simulink model "BatterySOHEstimation"  (R2024a)
settings: Solver=VariableStepAuto  StartTime=0.0  StopTime=10*10000  FixedStep=Ts  RelTol=1e-3  EnableMultiTasking=on
PreLoadFcn:
  | BatterySOHEstimationData;
values from neighbouring files (symbols this model uses):
  R = 0.05    [BatterySOHEstimationData.m]
  R00 = 0.008    [BatterySOHEstimationData.m]
  R0_mat = [.0117, .0085, .009; .011, .0085, .009;     .0114, .0087, .0092; .0107, .0082, .0088; .0107, .0083, .0091;     .0113, .0085, .0089; .0116, .0085, .0089]    [BatterySOHEstimationData.m]
  SOC0 = initialSOC    (= 0.1)    [BatterySOHEstimationData.m]
  Ts = 1    [BatterySOHEstimationData.m]
libraries: fl_lib x8, nesl_utility x5, simulink x3, BatteryEstimators x2, batteryecm_lib x1
CloseFcn:
  | try
  |     close(h1_BatterySOHEstimation)
  | catch
  | end
  | 
  | clear h1_BatterySOHEstimation
  | 
  | clear BatterySOHEstimationSimlog
  | clear BatterySOHEstimationLogsout
  | 
  | clear AH SOC_vec T_vec R0_mat R1_mat tau1_mat
  | clear V0_mat Q R P0 initialSOC SOC0 R00 Ts
  | clear cell_area h_conv thermal_mass
Description:
  | Battery State-of-Health Estimation
settings Model: Creator=The MathWorks, Inc.  LastModifiedBy=Carlos
settings SolverCC: AlgebraicLoopSolver=TrustRegion  AutoInsertRateTranBlk=on  MaxZcPerStep=1
settings DataIOCC: MaxDataPoints=370000  ReturnWorkspaceOutputs=off  SignalLoggingName=BatterySOHEstimationLogsout
settings OptimizationCC: ReuseModelBlockBuffer=off  LifeSpan=inf
settings DebuggingCC: UnconnectedInputMsg=warning  UnconnectedOutputMsg=warning  UnconnectedLineMsg=warning  SFUnexpectedBacktrackingDiag=warning  SFNoUnconditionalDefaultTransitionDiag=warning  SFExecutionAtInitializationDiag=none  ArithmeticOperatorsInVariantConditions=warning
settings ModelReferenceCC: EnableRefExpFcnMdlSchedulingChecks=on
settings SFSimCC: SimUseLocalCustomCode=off  CustomCodeUndefinedFunction=UseInterfaceOnly
settings RTWCC: RTWUseLocalCustomCode=off  GPUComputeCapability=3.5  DLArmComputeVersion=19.05
settings CodeAppCC: StateflowObjectComments=on
settings GRTTargetCC: TargetLangStandard=C89/C90 (ANSI)
settings ConfigComp: CovMetricSettings=dw  CovSaveCumulativeToWorkspaceVar=on  CovSaveSingleToWorkspaceVar=on  CovExternalEMLEnable=off
settings SimscapeCC: SimscapeLogType=all  SimscapeLogSimulationStatistics=on  SimscapeLogName=BatterySOHEstimationSimlog  SimscapeLogDataHistory=370000

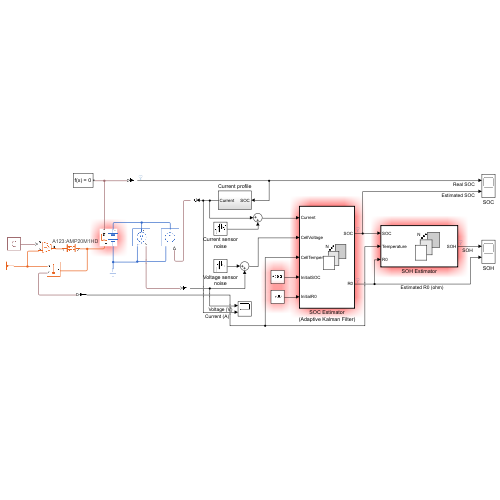
[thumbnail: Simulink's stored preview of the top-level diagram]
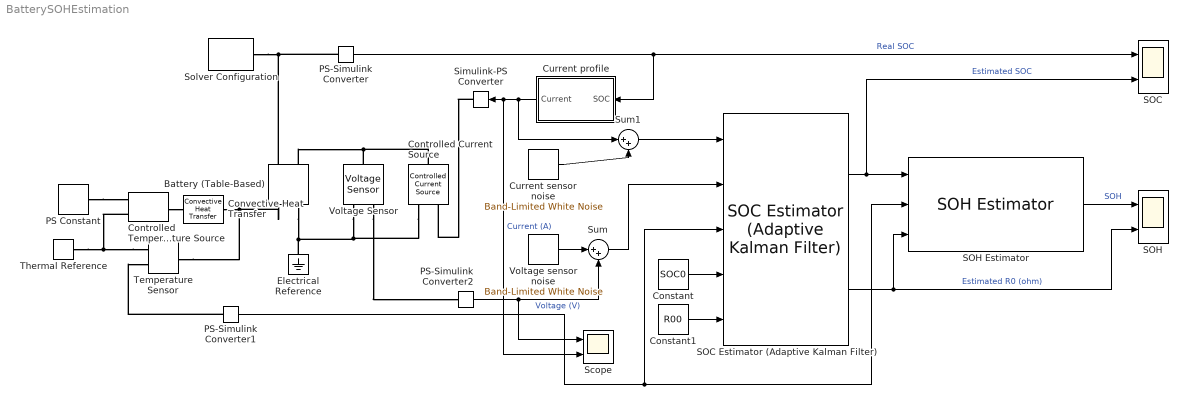
== system BatterySOHEstimation ==
  Battery (Table-Based) : batteryecm_lib/Battery (Table-Based)  Tag={'toolbox/physmod/battery/shared_library/m/batteryecm_lib_parts';'Battery__Table_Based_/A123/AMP20M1HD.xml'}  SOC_vec=SOC_vec  T_dependence=simscape.enum.tablebattery.temperature_dependence.yes  prm_dir=simscape.enum.tablebattery.prm_dir.noCurrentDirectionality  T_vec=T_vec K  V0_mat=V0_mat V  V0_vec=[2.93217 2.94263 2.95309 2.96355 2.97401 2.98447 2.99493 3.02455 3.05382 3.07377 3.08453 3.09529 3.09916 3.10271 3.10625 3.1098 3.11335 3.11689 3.12044 3.13089 3.13795 3.14459 3.14961 3.15451 3.15932 3.16324 3.16716 3.17063 3.17297 3.17544 3.17798 3.18052 3.18295 3.18533 3.18771 3.19009 3.19215 3.19403 3.1959 3.19777 3.1998 3.20198 3.20371 3.20501 3.20619 3.20738 3.20856 3.20974 3.21092 3.2121 3.21329 3.21447 3.21565 3.21672 3.21787 3.21904 3.22021 3.22139 3.22256 3.22374 3.22492 3.2261 3.22728 3.22847 3.22965 3.23083 3.23201 3.23319 3.23437 3.23552 3.23652 3.23778 3.23909 3.24045 3.24217 3.2439 3.24563 3.24736 3.24909 3.25082 3.25255 3.25428 3.256 3.25774 3.25951 3.26116 3.26238 3.26307 3.26352 3.26396 3.26441 3.26485 3.2653 3.26593 3.26612 3.26743 3.26879 3.27596 3.2842 3.30299 3.33677] V  V_range=[1.8 Inf] V  R0_mat=R0_mat Ohm  R0_vec=[0.00349 0.0033 0.00311 0.00292 0.00272 0.00253 0.00235 0.00233 0.00235 0.00232 0.00223 0.00214 0.00205 0.00196 0.00187 0.00181 0.00175 0.00169 0.00164 0.00167 0.00168 0.00168 0.00168 0.00168 0.00167 0.00167 0.00167 0.00167 0.00166 0.00165 0.00164 0.00164 0.00163 0.00163 0.00162 0.00162 0.00161 0.0016 0.00159 0.00159 0.00158 0.00158 0.00158 0.00157 0.00156 0.00156 0.00155 0.00154 0.00154 0.00153 0.00153 0.00152 0.00151 0.00151 0.0015 0.0015 0.0015 0.00149 0.00149 0.00149 0.00148 0.00148 0.00148 0.00147 0.00147 0.00147 0.00147 0.00146 0.00146 0.00146 0.00145 0.00146 0.00146 0.00147 0.00147 0.00148 0.00149 0.0015 0.0015 0.00151 0.00152 0.00153 0.00153 0.00154 0.00155 0.00155 0.00156 0.00155 0.00154 0.00153 0.00152 0.00151 0.0015 0.00148 0.00144 0.0014 0.00137 0.00136 0.00131 0.00127 0.00104] Ohm  R0_dis_mat=[.0117, .0085, .009; .011, .0085, .009; .0114, .0087, .0092; .0107, .0082, .0088; .0107, .0083, .0091; .0113, .0085, .0089; .0116, .0085, .0089] % Parameter not set Ohm  R0_dis_vec=[.0085, .0085, .0087, .0082, .0083, .0085, .0085] % Parameter not set Ohm  R0_ch_mat=[.0117, .0085, .009; .011, .0085, .009; .0114, .0087, .0092; .0107, .0082, .0088; .0107, .0083, .0091; .0113, .0085, .0089; .0116, .0085, .0089] % Parameter not set Ohm  R0_ch_vec=[.0085, .0085, .0087, .0082, .0083, .0085, .0085] % Parameter not set Ohm  AH=AH hr*A  prm_leak=simscape.enum.tablebattery.prm_leak.disabled  Rleak_vec=[8000, 7000, 6000] % Parameter not set Ohm  Rleak=7e3 % Parameter not set Ohm  extrapolation_option=simscape.enum.extrapolation.nearest  SOC_port=simscape.enum.tablebattery.enable.yes  prm_dyn=simscape.enum.tablebattery.prm_dyn.rc1  R1_mat=R1_mat Ohm  R1_vec=[.0029, .0024, .0026, .0016, .0023, .0018, .0017] % Parameter not set Ohm  tau1_mat=tau1_mat s  tau1_vec=[36, 45, 105, 29, 77, 33, 39] % Parameter not set s  R2_mat=[.0109, .0029, .0013; .0069, .0024, .0012; .0047, .0026, .0013; .0034, .0016, .001; .0033, .0023, .0014; .0033, .0018, .0011; .0028, .0017, .0011] % Parameter not set Ohm  R2_vec=[.0029, .0024, .0026, .0016, .0023, .0018, .0017] % Parameter not set Ohm  tau2_mat=[20, 36, 39; 31, 45, 39; 109, 105, 61; 36, 29, 26; 59, 77, 67; 40, 33, 29; 25, 39, 33] % Parameter not set s  tau2_vec=[36, 45, 105, 29, 77, 33, 39] % Parameter not set s  R3_mat=[.0109, .0029, .0013; .0069, .0024, .0012; .0047, .0026, .0013; .0034, .0016, .001; .0033, .0023, .0014; .0033, .0018, .0011; .0028, .0017, .0011] % Parameter not set Ohm  R3_vec=[.0029, .0024, .0026, .0016, .0023, .0018, .0017] % Parameter not set Ohm  tau3_mat=[20, 36, 39; 31, 45, 39; 109, 105, 61; 36, 29, 26; 59, 77, 67; 40, 33, 29; 25, 39, 33] % Parameter not set s  tau3_vec=[36, 45, 105, 29, 77, 33, 39] % Parameter not set s  R4_mat=[.0109, .0029, .0013; .0069, .0024, .0012; .0047, .0026, .0013; .0034, .0016, .001; .0033, .0023, .0014; .0033, .0018, .0011; .0028, .0017, .0011] % Parameter not set Ohm  R4_vec=[.0029, .0024, .0026, .0016, .0023, .0018, .0017] % Parameter not set Ohm  tau4_mat=[20, 36, 39; 31, 45, 39; 109, 105, 61; 36, 29, 26; 59, 77, 67; 40, 33, 29; 25, 39, 33] % Parameter not set s  tau4_vec=[36, 45, 105, 29, 77, 33, 39] % Parameter not set s  R5_mat=[.0109, .0029, .0013; .0069, .0024, .0012; .0047, .0026, .0013; .0034, .0016, .001; .0033, .0023, .0014; .0033, .0018, .0011; .0028, .0017, .0011] % Parameter not set Ohm  R5_vec=[.0029, .0024, .0026, .0016, .0023, .0018, .0017] % Parameter not set Ohm  tau5_mat=[20, 36, 39; 31, 45, 39; 109, 105, 61; 36, 29, 26; 59, 77, 67; 40, 33, 29; 25, 39, 33] % Parameter not set s  tau5_vec=[36, 45, 105, 29, 77, 33, 39] % Parameter not set s  prm_fade=simscape.enum.tablebattery.prm_fade.tableNandT  N0=100 % Parameter not set  dV0=0 % Parameter not set  dR0=0 % Parameter not set  dAH=0 % Parameter not set  dRleak=0 % Parameter not set  dR1=0 % Parameter not set  dR2=0 % Parameter not set  dR3=0 % Parameter not set  dR4=0 % Parameter not set  dR5=0 % Parameter not set  N0vec=N0vec  Tfadevec=Tfadevec K  dV0vec=[0 -0.3227 -0.6453 -0.9509 -1.1187 -1.2594 -1.4 -1.5407 -1.6219 -1.683 -1.7439 -1.8049 -1.8602 -1.9134 -1.9665 -2.0196 -2.0441 -2.0544 -2.0647 -2.075 -2.085 -2.0949 -2.1048 -2.1146 -2.1183 -2.1198 -2.1212 -2.1226 -2.1259 -2.1303 -2.1347 -2.1391 -2.1431 -2.1462 -2.1493 -2.1524 -2.1556 -2.1591 -2.1625 -2.166 -2.1695 -2.1729 -2.1764 -2.1798 -2.1833 -2.1867 -2.1902 -2.1936 -2.197 -2.2002 -2.2034 -2.2067 -2.2106 -2.2156 -2.2206 -2.2256 -2.2316 -2.2405 -2.2493 -2.2582 -2.2676 -2.2798 -2.292 -2.3042 -2.3164 -2.3294 -2.3424 -2.3556 -2.3688 -2.3818 -2.3947 -2.4077 -2.4207 -2.4336 -2.4465 -2.4594 -2.4722 -2.485 -2.4978 -2.5106 -2.5233 -2.5361 -2.5489 -2.5617 -2.5745 -2.5872 -2.5999 -2.6126 -2.6253 -2.6381 -2.6508 -2.6635 -2.6765 -2.6898 -2.703 -2.7163 -2.7295 -2.7428 -2.756 -2.7693]  dR0vec=[0 0 0 0 0 0 0 0 0 0 0 0 0 0 0 0 0 0 0 0 0 0 0 0 0 0 0 0 0 0 0 0 0 0 0 0 0 0 0 0 0 0 0 0 0 0 0 0 0 0 0 0 0 0 0 0 0 0 0 0 0 0 0 0 0 0 0 0 0 0 0 0 0 0 0 0 0 0 0 0 0 0 0 0 0 0 0 0 0 0 0 0 0 0 0 0 0 0 0 0] % Parameter assumed  dAHvec=[0 -0.319 -0.638 -0.939 -1.189 -1.439 -1.688 -1.938 -2.188 -2.435 -2.682 -2.93 -3.177 -3.424 -3.671 -3.918 -4.169 -4.421 -4.673 -4.925 -5.177 -5.429 -5.681 -5.933 -6.185 -6.437 -6.683 -6.917 -7.152 -7.386 -7.621 -7.855 -8.09 -8.324 -8.558 -8.793 -9.033 -9.292 -9.551 -9.809 -10.068 -10.327 -10.586 -10.845 -11.104 -11.363 -11.622 -11.88 -12.132 -12.374 -12.616 -12.857 -13.099 -13.341 -13.582 -13.824 -14.066 -14.307 -14.549 -14.791 -15.035 -15.281 -15.526 -15.772 -16.017 -16.263 -16.508 -16.757 -17.007 -17.256 -17.506 -17.755 -18.005 -18.254 -18.504 -18.752 -18.999 -19.246 -19.493 -19.74 -19.986 -20.233 -20.48 -20.727 -20.973 -21.219 -21.464 -21.71 -21.955 -22.201 -22.446 -22.692 -22.943 -23.199 -23.455 -23.711 -23.966 -24.222 -24.478 -24.733]  dRleakvec=[0, 0, 0, 0] % Parameter not set  dR1vec=[0, 0, 0, 0] % Parameter not set  dR2vec=[0, 0, 0, 0] % Parameter not set  dR3vec=[0, 0, 0, 0] % Parameter not set  dR4vec=[0, 0, 0, 0] % Parameter not set  dR5vec=[0, 0, 0, 0] % Parameter not set  dV0mat=dV0mat  dR0mat=dR0mat  dAHmat=dAHmat  dRleakmat=[0, 0; 0, 0; 0, 0; 0, 0] % Parameter not set  dR1mat=dR1mat  dR2mat=[0, 0; 0, 0; 0, 0; 0, 0] % Parameter not set  dR3mat=[0, 0; 0, 0; 0, 0; 0, 0] % Parameter not set  dR4mat=[0, 0; 0, 0; 0, 0; 0, 0] % Parameter not set  dR5mat=[0, 0; 0, 0; 0, 0; 0, 0] % Parameter not set  prm_age_modeling=simscape.enum.tablebattery.prm_age_modeling.tableTandTime  storage_dt_age_vec=storage_dt_age_vec d  storage_T_age_vec=storage_T_age_vec K  prm_age_OCV=simscape.enum.tablebattery.prm_age_OCV.OCV  OCV_age=0.9 % Parameter not set  SOC_age=0.6 % Parameter not set  prm_age_resistance=simscape.enum.tablebattery.prm_age.disabled  OCV_scaling_age_resistance=2.2134e6 % Parameter not set  OCV_offset_age_resistance=1.632e6 % Parameter not set  temp_exp_age_resistance=0.515833569 % Parameter not set V  t_exp_age_resistance=0.75 % Parameter not set  T_age_vec_resistance=[273.15, 298.15, 323.15] % Parameter not set K  dt_age_vec_resistance=[0, 90, 180, 270] % Parameter not set d  dR0_age_vec=[0, 0, 0] % Parameter not set  t_meas_dR0_age=100 % Parameter not set d  dR0_age_mat=[0, 0, 0; 0, 0, 0; 0, 0, 0; 0, 0, 0] % Parameter not set  prm_age_capacity=simscape.enum.tablebattery.prm_age.enabled  OCV_scaling_age_capacity=1.5097e07 % Parameter not set  OCV_offset_age_capacity=8.3625e06 % Parameter not set  temp_exp_age_capacity=0.6011 % Parameter not set V  t_exp_age_capacity=0.75 % Parameter not set  T_age_vec_capacity=T_age_vec_capacity K  dt_age_vec_capacity=dt_age_vec_capacity d  dAH_age_vec=[0, 0, 0] % Parameter not set  t_meas_dAH_age=100 % Parameter not set d  dAH_age_mat=dAH_age_mat  thermal_port=simscape.enum.thermaleffects.model  temperature=298.15 % Parameter not set K  thermal_mass=446.4 % Parameter assumed J/K  i_specify=on  i_priority=None  i=i A  i_nominal_specify=off  i_nominal_value=1  i_nominal_unit=A  v_specify=on  v_priority=None  v=v V  v_nominal_specify=on  v_nominal_value=v_nominal_value  v_nominal_unit=V  stateOfCharge_specify=on  stateOfCharge_priority=High  stateOfCharge=initialSOC  stateOfCharge_nominal_specify=on  stateOfCharge_nominal_value=finalSOC  stateOfCharge_nominal_unit=1  num_cycles_specify=on  num_cycles_priority=High  num_cycles=num_cycles  num_cycles_nominal_specify=on  num_cycles_nominal_value=num_cycles_nominal_value  num_cycles_nominal_unit=1  cell_temperature_specify=on  cell_temperature_priority=High  cell_temperature=cell_temperature K  cell_temperature_nominal_specify=off  cell_temperature_nominal_value=1  cell_temperature_nominal_unit=K
      settings: AttributesFormatString=A123:AMP20M1HD
  Constant : Constant  Value=SOC0
  Constant1 : Constant  Value=R00
  Controlled Temperature Source : fl_lib/Thermal/Thermal Sources/Controlled Temperature Source
  Controlled Current Source : fl_lib/Electrical/Electrical Sources/Controlled Current Source
  Convective Heat Transfer : fl_lib/Thermal/Thermal Elements/Convective Heat Transfer  thermal_type=foundation.enum.constant_variable.constant  area=0.1019 m^2  heat_tr_coeff=5 W/(K*m^2)  min_heat_tr_coeff=1e-3 W/(K*m^2)  T_specify=off  T_priority=None  T=0 K  T_nominal_specify=off  T_nominal_value=1  T_nominal_unit=K  Q_specify=off  Q_priority=None  Q=0 W  Q_nominal_specify=off  Q_nominal_value=1  Q_nominal_unit=W
  Current profile : Subsystem
  Current sensor noise : simulink/Sources/Band-Limited White Noise  Cov=1e-3  Ts=1  seed=1
  Electrical Reference : fl_lib/Electrical/Electrical Elements/Electrical Reference
  PS Constant : fl_lib/Physical Signals/Sources/PS Constant  constant=292.15 K
  PS-Simulink Converter : nesl_utility/PS-Simulink Converter  PhysicalDomain=network_engine_domain  SubClassName=ps_output  LeftPortType=input  RightPortType=output  PseudoPeriodic=off  Frequencies=[]  VectorFormat=inherit  Unit=inherit  AffineConversion=off
  PS-Simulink Converter1 : nesl_utility/PS-Simulink Converter  PhysicalDomain=network_engine_domain  SubClassName=ps_output  LeftPortType=input  RightPortType=output  PseudoPeriodic=off  Frequencies=[]  VectorFormat=inherit  Unit=inherit  AffineConversion=off
  PS-Simulink Converter2 : nesl_utility/PS-Simulink Converter  PhysicalDomain=network_engine_domain  SubClassName=ps_output  LeftPortType=input  RightPortType=output  PseudoPeriodic=off  Frequencies=[]  VectorFormat=inherit  Unit=inherit  AffineConversion=off
  SOC : Scope  NumInputPorts=2
  SOC Estimator (Adaptive Kalman Filter) : BatteryEstimators/SOC Estimator (Adaptive Kalman Filter)  CurrentInputPartition=off  filterType=Unscented Kalman filter  alpha=1  beta=2  kappa=0  Q=Q  Q_2RC=|  R=R  P0=P0  P0_2RC="[1e-5 0 0 0; 0 1 0 0;0 0  1 0; 0 0 0 1e-5]"  Ts=Ts  chargeDynamics=One time-constant dynamics  SOC_vec=SOC_vec  T_vec=T_vec  R1_mat=R1_mat  tau1_mat=tau1_mat  R2_mat=[.0109, .0029, .0013; .0069, .0024, .0012; .0047, .0026, .0013; .0034, .0016, .001; .0033, .0023, .0014; .0033, .0018, .0011; .0028, .0017, .0011]  tau2_mat=[20, 36, 39; 31, 45, 39; 109, 105, 61; 36, 29, 26; 59, 77, 67; 40, 33, 29; 25, 39, 33]  V0_mat=V0_mat  AH=AH
      | [1e-6 0 0 0;
      | 0 1e-6 0 0;0 0 1e-6 0;0 0 0 1e-6]
  SOH : Scope  NumInputPorts=2
  SOH Estimator : BatteryEstimators/SOH Estimator  SOC_vec=SOC_vec  T_vec=T_vec  R0_new_mat=R0_mat  R0_EOL_mat=R0_mat*3
  Scope : Scope  NumInputPorts=2
  Simulink-PS Converter : nesl_utility/Simulink-PS Converter  PhysicalDomain=network_engine_domain  SubClassName=ps_input  LeftPortType=input  RightPortType=output  PseudoPeriodic=off  Frequencies=[]  NoiseDistribution=none  NoiseParameters=[]  Unit=1  AffineConversion=off  FilteringAndDerivatives=provide  SimscapeFilterOrder=1  InputFilterTimeConstant=0.001  UdotUserProvided=0
  Solver Configuration : nesl_utility/Solver Configuration  PhysicalDomain=network_engine_domain  SubClassName=solver  LeftPortType=input  RightPortType=generic  Tones=[]  Harmonics=[]  SimulateNoise=off  Profile=off  UseLocalSampling=off  EnableSwitchedLinearOptims=on  FrequencyDomain=off  UseCCode=off  RelTol=0.001  AbsTol=0.001  MinStep=1e-09  ToWorkspace=off  RevertToSquareIcSolve=off  NumHomotopyIterations=100  PhasorMode=off  PhasorModeNumHarmonics=1  ConsistencySolver=NEWTON_XTOL_AFTER_FTOL  IndexReductionMethod=DerivativeReplacement  DoDC=off  ResidualTolerance=1e-09  ConsistencyTolSource=GLOBAL  ConsistencyAbsTol=0.001  ConsistencyRelTol=0.001  ConsistencyTolFactor=0.001  UseLocalSolver=off  LocalSolverChoice=NE_BACKWARD_EULER_ADVANCER  ResolveIndetEquations=on  FunctionEvalNumThread=1  LocalSolverSampleTime=0.001  DoFixedCost=off  MaxNonlinIter=3  MaxModeIter=2  ComputeImpulses=off  ImpulseIterations=2  LinearAlgebra=auto  LinearAlgebraNumThread=0  EquationFormulation=NE_TIME_EF  DelaysMemoryBudget=1024  AutomaticFiltering=on  FilteringTimeConstant=0.001  PartitionStorageMethod=AS_NEEDED  PartitionMemoryBudget=1024  PartitionMethod=ROBUST  MultibodyUseLocalSolver=off  MultibodyLocalSolverChoice=ODE1  MultibodyLocalSolverSampleTime=0.001
  Sum : Sum  Inputs=|++
  Sum1 : Sum  Inputs=|++
  Temperature Sensor : fl_lib/Thermal/Thermal Sensors/Temperature Sensor  temperature_measure=foundation.enum.MeasurementReference.difference
  Thermal Reference : fl_lib/Thermal/Thermal Elements/Thermal Reference
  Voltage Sensor : fl_lib/Electrical/Electrical Sensors/Voltage Sensor
  Voltage sensor noise : simulink/Sources/Band-Limited White Noise  Cov=1e-3  Ts=1  seed=23341
  wires:
  Sum1/1 -> SOC Estimator (Adaptive Kalman Filter)/1
  Sum/1 -> SOC Estimator (Adaptive Kalman Filter)/2
  PS-Simulink Converter1/1 -> SOH Estimator/2, SOC Estimator (Adaptive Kalman Filter)/3
  Constant/1 -> SOC Estimator (Adaptive Kalman Filter)/4
  Constant1/1 -> SOC Estimator (Adaptive Kalman Filter)/5
  SOC Estimator (Adaptive Kalman Filter)/1 -> SOH Estimator/1, SOC/2  "Estimated SOC"
  SOC Estimator (Adaptive Kalman Filter)/2 -> SOH/2, SOH Estimator/3  "Estimated R0 (ohm)"
  Current profile/1(Current) -> Sum1/1, Scope/2, Simulink-PS Converter/1  "Current (A)"
  PS-Simulink Converter/1 -> Current profile/1(SOC), SOC/1  "Real SOC"
  SOH Estimator/1 -> SOH/1  "SOH"
  Voltage sensor noise/1 -> Sum/1
  Current sensor noise/1 -> Sum1/2
  PS-Simulink Converter2/1 -> Scope/1, Sum/2  "Voltage (V)"
  connections:
  PS-Simulink Converter/LConn1 -- Battery (Table-Based)/LConn2 -- Solver Configuration/RConn1
  Electrical Reference/LConn1 -- Battery (Table-Based)/RConn1 -- Controlled Current Source/RConn2 -- Voltage Sensor/RConn2
  Voltage Sensor/LConn1 -- Battery (Table-Based)/LConn1 -- Controlled Current Source/LConn1
  Simulink-PS Converter/RConn1 -- Controlled Current Source/RConn1
  Voltage Sensor/RConn1 -- PS-Simulink Converter2/LConn1
  Temperature Sensor/LConn1 -- Battery (Table-Based)/RConn2 -- Convective Heat Transfer/LConn1
  Temperature Sensor/RConn1 -- Thermal Reference/LConn1 -- Controlled Temperature Source/RConn2
  Controlled Temperature Source/LConn1 -- Convective Heat Transfer/RConn1
  PS-Simulink Converter1/LConn1 -- Temperature Sensor/RConn2
  PS Constant/RConn1 -- Controlled Temperature Source/RConn1

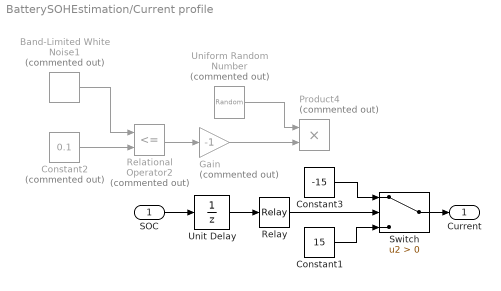
== system BatterySOHEstimation/Current profile ==
  SOC : Inport
  Band-Limited White Noise1 : simulink/Sources/Band-Limited White Noise  Commented=on  Cov=1  Ts=50  seed=[23341]
  Constant1 : Constant  Value=15
  Constant2 : Constant  Commented=on  Value=0.1
  Constant3 : Constant  Value=-15
  Gain : Gain  Commented=on  Gain=-1
  Product4 : Product  Commented=on
  Relational Operator2 : RelationalOperator  Commented=on  Operator=<=  OutDataTypeStr=boolean  RndMeth=Simplest  InputSameDT=off
  Relay : Relay  OnSwitchValue=0.9  OffSwitchValue=0.3  OffOutputValue=-1
  Switch : Switch  Criteria=u2 > Threshold  SaturateOnIntegerOverflow=off  InputSameDT=off
  Uniform Random Number : UniformRandomNumber  Commented=on  Minimum=5  Maximum=55  SampleTime=100
  Unit Delay : UnitDelay  SampleTime=Ts  HasFrameUpgradeWarning=on
  Current : Outport
  wires:
  Constant2/1 -> Relational Operator2/2
  Relational Operator2/1 -> Gain/1
  Gain/1 -> Product4/2
  Band-Limited White Noise1/1 -> Relational Operator2/1
  Uniform Random Number/1 -> Product4/1
  Switch/1 -> Current/1
  Unit Delay/1 -> Relay/1
  Relay/1 -> Switch/2
  Constant1/1 -> Switch/3
  SOC/1 -> Unit Delay/1
  Constant3/1 -> Switch/1
